simulink model "good_version_model4_1"  (R2015a)
settings: Solver=ode45  SolverMode=SingleTasking  StartTime=0.0  StopTime=80  RelTol=1e-3
libraries: simulink x2
settings Model: CovMetricSettings=dwe  CovHtmlReporting=off  covSaveCumulativeToWorkspaceVar=off  CovSaveSingleToWorkspaceVar=off  CovExternalEMLEnable=on  Creator=L1.3-20  LastModifiedBy=Kornel
settings DataIOCC: LimitDataPoints=off  SaveFormat=Dataset
settings DebuggingCC: SFUnexpectedBacktrackingDiag=error  SFNoUnconditionalDefaultTransitionDiag=error
settings HardwareCC: ProdBitPerPointer=64  ProdLargestAtomicFloat=Float  ProdIntDivRoundTo=Zero  ProdEndianess=LittleEndian  ProdHWDeviceType=Specified
settings ModelReferenceCC: PropagateSignalLabelsOutOfModel=on
settings GRTTargetCC: TargetLangStandard=C99 (ISO)  GeneratePreprocessorConditionals=Use local settings

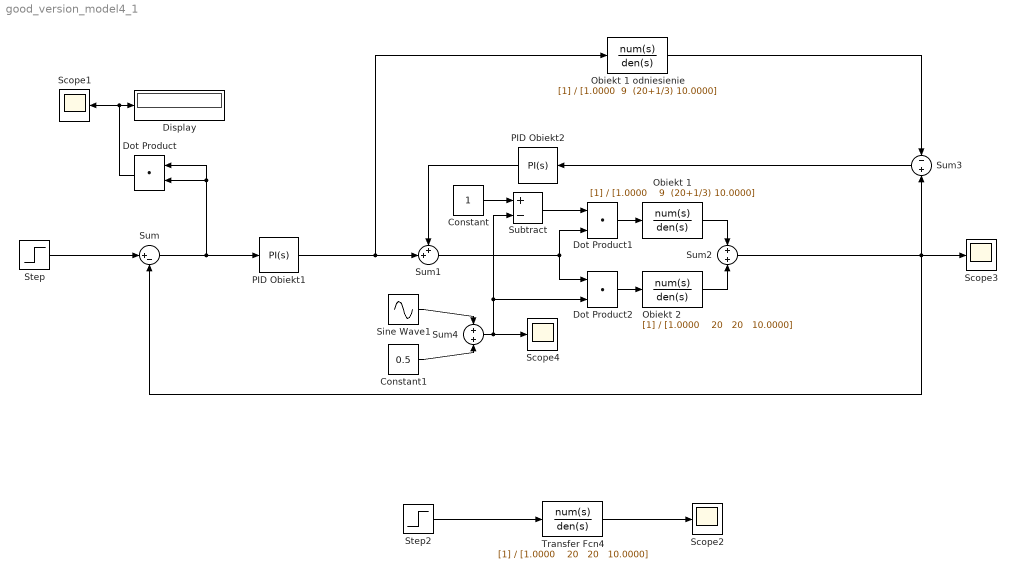
== system good_version_model4_1 ==
  Constant : Constant
  Constant1 : Constant  Value=0.5
  Display : Display
  Dot Product : DotProduct  InputSameDT=on  OutDataTypeStr=Inherit: Inherit via internal rule
  Dot Product1 : DotProduct  InputSameDT=on  OutDataTypeStr=Inherit: Inherit via internal rule
  Dot Product2 : DotProduct  InputSameDT=on  OutDataTypeStr=Inherit: Inherit via internal rule
  Obiekt 1 : TransferFcn  Denominator="[1.0000    9  (20+1/3) 10.0000]"
  Obiekt 1 odniesienie : TransferFcn  Denominator="[1.0000  9  (20+1/3) 10.0000]"
  Obiekt 2 : TransferFcn  Denominator="[1.0000    20   20   10.0000]"
  PID Obiekt1 : simulink/Continuous/PID Controller  Controller=PI  TimeDomain=Continuous-time  SampleTime=-1  IntegratorMethod=Forward Euler  FilterMethod=Forward Euler  Form=Parallel  UseFilter=on  ControllerParametersSource=internal  P=0  I=2  D=6.24481448440131  N=131.561600216023  InitialConditionSource=internal  InitialConditionForIntegrator=0  InitialConditionForFilter=0  ExternalReset=none  LimitOutput=off  UpperSaturationLimit=inf  LowerSaturationLimit=-inf  LinearizeAsGain=on  AntiWindupMode=none  Kb=1  TrackingMode=off  Kt=1  PParamMin=[]  PParamMax=[]  IParamMin=[]  IParamMax=[]  DParamMin=[]  DParamMax=[]  NParamMin=[]  NParamMax=[]  KbParamMin=[]  KbParamMax=[]  KtParamMin=[]  KtParamMax=[]  POutMin=[]  POutMax=[]  IOutMin=[]  IOutMax=[]  DOutMin=[]  DOutMax=[]  NOutMin=[]  NOutMax=[]  KbOutMin=[]  KbOutMax=[]  KtOutMin=[]  KtOutMax=[]  IntegratorOutMin=[]  IntegratorOutMax=[]  FilterOutMin=[]  FilterOutMax=[]  SumOutMin=[]  SumOutMax=[]  SumI1OutMin=[]  SumI1OutMax=[]  SumI2OutMin=[]  SumI2OutMax=[]  SumI3OutMin=[]  SumI3OutMax=[]  SumDOutMin=[]  SumDOutMax=[]  SaturationOutMin=[]  SaturationOutMax=[]  IntegratorContinuousStateAttributes=''  IntegratorStateMustResolveToSignalObject=off  IntegratorRTWStateStorageClass=Auto  FilterContinuousStateAttributes=''  FilterStateMustResolveToSignalObject=off  FilterRTWStateStorageClass=Auto  DifferentiatorICPrevScaledInput=0  DifferentiatorOutMin=[]  DifferentiatorOutMax=[]
  PID Obiekt2 : simulink/Continuous/PID Controller  Controller=PI  TimeDomain=Continuous-time  SampleTime=-1  IntegratorMethod=Forward Euler  FilterMethod=Forward Euler  Form=Parallel  UseFilter=on  ControllerParametersSource=internal  P=-2.7  I=-4.7  D=6.24481448440131  N=131.561600216023  InitialConditionSource=internal  InitialConditionForIntegrator=0  InitialConditionForFilter=0  ExternalReset=none  LimitOutput=off  UpperSaturationLimit=inf  LowerSaturationLimit=-inf  LinearizeAsGain=on  AntiWindupMode=none  Kb=1  TrackingMode=off  Kt=1  PParamMin=[]  PParamMax=[]  IParamMin=[]  IParamMax=[]  DParamMin=[]  DParamMax=[]  NParamMin=[]  NParamMax=[]  KbParamMin=[]  KbParamMax=[]  KtParamMin=[]  KtParamMax=[]  POutMin=[]  POutMax=[]  IOutMin=[]  IOutMax=[]  DOutMin=[]  DOutMax=[]  NOutMin=[]  NOutMax=[]  KbOutMin=[]  KbOutMax=[]  KtOutMin=[]  KtOutMax=[]  IntegratorOutMin=[]  IntegratorOutMax=[]  FilterOutMin=[]  FilterOutMax=[]  SumOutMin=[]  SumOutMax=[]  SumI1OutMin=[]  SumI1OutMax=[]  SumI2OutMin=[]  SumI2OutMax=[]  SumI3OutMin=[]  SumI3OutMax=[]  SumDOutMin=[]  SumDOutMax=[]  SaturationOutMin=[]  SaturationOutMax=[]  IntegratorContinuousStateAttributes=''  IntegratorStateMustResolveToSignalObject=off  IntegratorRTWStateStorageClass=Auto  FilterContinuousStateAttributes=''  FilterStateMustResolveToSignalObject=off  FilterRTWStateStorageClass=Auto  DifferentiatorICPrevScaledInput=0  DifferentiatorOutMin=[]  DifferentiatorOutMax=[]
  Scope{1..4} (4 alike) : Scope
      Scope1 settings: YMin=-0.125  YMax=1.125
      Scope2 settings: YMin=-0.1735  YMax=1.56148  SaveName=ScopeData2
      Scope3 settings: YMin=-0.125  YMax=1.125  SaveName=ScopeData3
      Scope4 settings: YMin=-0.125  YMax=1.125
  Sine Wave1 : Sin  Amplitude=0.5  Frequency=10  SampleTime=0
  Step : Step  SampleTime=0
  Step2 : Step  Time=5  SampleTime=0
  Subtract : Sum  Inputs=+-
  Sum : Sum  Inputs=|+-
  Sum1 : Sum  Inputs=++|
  Sum2 : Sum  Inputs=+|+
  Sum3 : Sum  Inputs=-|+
  Sum4 : Sum  Inputs=+|+
  Transfer Fcn4 : TransferFcn  Denominator="[1.0000    20   20   10.0000]"
  wires:
  Sum/1 -> Dot Product/2, Dot Product/1, PID Obiekt1/1
  Sum2/1 -> Sum/2, Scope3/1, Sum3/2
  Step/1 -> Sum/1
  Dot Product/1 -> Scope1/1, Display/1
  PID Obiekt1/1 -> Obiekt 1 odniesienie/1, Sum1/2
  Sum3/1 -> PID Obiekt2/1
  PID Obiekt2/1 -> Sum1/1
  Obiekt 1 odniesienie/1 -> Sum3/1
  Step2/1 -> Transfer Fcn4/1
  Transfer Fcn4/1 -> Scope2/1
  Obiekt 1/1 -> Sum2/1
  Obiekt 2/1 -> Sum2/2
  Dot Product2/1 -> Obiekt 2/1
  Dot Product1/1 -> Obiekt 1/1
  Sum1/1 -> Dot Product2/1, Dot Product1/2
  Subtract/1 -> Dot Product1/1
  Constant/1 -> Subtract/1
  Constant1/1 -> Sum4/2
  Sine Wave1/1 -> Sum4/1
  Sum4/1 -> Scope4/1, Dot Product2/2, Subtract/2
